simulink model "simu_py"  (R2025b)
settings: Solver=ode8  StartTime=0.0  StopTime=5  FixedStep=0.001  RelTol=1e-3
libraries: autolibshared x1
(part 2 of 2)

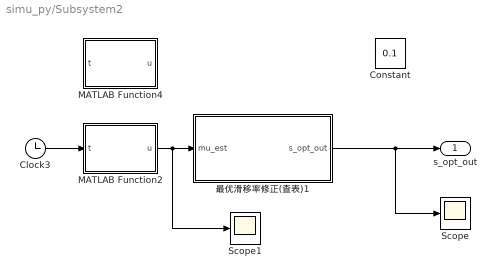
== system simu_py/Subsystem2 ==
  Clock3 : Clock
  Constant : Constant  Value=0.1
  MATLAB Function2 : MATLAB Function  TreatAsAtomicUnit=on
  MATLAB Function4 : MATLAB Function  TreatAsAtomicUnit=on
  Scope : Scope
      settings: ActiveDisplayYMinimum=0.051875  ActiveDisplayYMaximum=0.183125  DataLoggingVariableName=lambda_ref  DataLoggingSaveFormat=Array
  Scope1 : Scope
      settings: DataLoggingVariableName=mu_rel  DataLoggingSaveFormat=Array
  最优滑移率修正(查表)1 : MATLAB Function  TreatAsAtomicUnit=on
  s_opt_out : Outport
  wires:
  最优滑移率修正(查表)1/1(s_opt_out) -> s_opt_out/1, Scope/1
  MATLAB Function2/1(u) -> Scope1/1, 最优滑移率修正(查表)1/1(mu_est)
  Clock3/1 -> MATLAB Function2/1(t)

== matlab function simu_py/MATLAB Function17 ==
  data: mu_init input; c1_out output; c2_out output; c3_out output
function [c1_out, c2_out, c3_out] = select_initial_c(mu_init)
% 输入：
%   mu_init - 初始路面峰值附着系数（标量）
% 输出：
%   c1_out, c2_out, c3_out - 表中差值最小行对应的 c1,c2,c3 （标量）
%
% 说明：表格格式为每行 [c1, c2, c3, s_opt, mu_max]

% 如果传入向量/数组，只取第一个元素（Simulink 通常给标量）
if isempty(mu_init)
    mu_init = 0;
end
mu_init = double(mu_init(1));

% ----- 参数表（硬编码） -----
% 每行： [c1, c2, c3, s_opt, mu_max]
tbl = [ ...
    0.05,  306.39, 0.001, 0.03, 0.05;
    0.195, 94.129, 0.065, 0.065,0.191;
    0.4,   33.712, 0.12,  0.13, 0.4;
    0.857, 33.822, 0.35,  0.14, 0.8;
    1.197, 25.166, 0.54,  0.16, 1.09;
    1.281, 23.992, 0.52,  0.17, 1.17];

% ----- 计算与返回 -----
mu_table = tbl(:,5);            % 表中 mu_max 列
[~, idx] = min(abs(mu_table - mu_init)); % 找到差值最小的行（首个最小）
c1_out = tbl(idx,1);
c2_out = tbl(idx,2);
c3_out = tbl(idx,3);
end

== matlab function simu_py/MATLAB Function3 ==
  data: t input; u output
function u = fcn(t)
if t<1.5
    u=1.09;
elseif t>=1.5&&t<2.8
    u = 0.15;
elseif t>=2.8&&t<3.3
    u = 0.9;
elseif t>=3.3&&t<4.1
    u = 0.45;
else
    u = 0.9;
end

== matlab function simu_py/MATLAB Function6 ==
  data: t input; u output
function u = fcn(t)
if t<1.5
    u=1.09;
elseif t>=1.5&&t<2.8
    u = 0.15;
elseif t>=2.8&&t<3.3
    u = 0.9;
elseif t>=3.3&&t<4.1
    u = 0.45;
else
    u = 0.9;
end

== matlab function simu_py/MATLAB Function7 ==
  settings: updateMethod=DISCRETE
  data: Fz input; Td_out output; mu input; omega input; lambda_k input; lambda_ref input
function Td_out = OnlineFmincon_block(Fz, mu, omega, lambda_k, lambda_ref)
% Called inside Simulink MATLAB Function block
coder.extrinsic('my_sqp_nmpc_fix_tyretran.m'); % wrapper is extrinsic (run in MATLAB workspace)

% persistent state for initial guess
persistent Td
if isempty(Td)
    Td = zeros(4,1)+1;
end

% Call the MATLAB wrapper (extrinsic) - all args numeric (no function handles)
Td_opt = my_sqp_nmpc_fix_tyretran(Td, Fz, mu, omega, lambda_k, lambda_ref);

% Td_opt will be returned as a MATLAB array (extrinsic) - may need conversion
% assign back, output
if ~isempty(Td_opt)
    Td = Td_opt;
end

Td_out = Td;
end

== matlab function simu_py/Subsystem2/MATLAB Function2 ==
  data: t input; u output
function u = fcn(t)
if t<1.5
    u=1.09;
elseif t>=1.5&&t<2.8
    u = 0.15;
elseif t>=2.8&&t<3.3
    u = 0.9;
elseif t>=3.3&&t<4.1
    u = 0.45;
else
    u = 0.9;
end

== matlab function simu_py/Subsystem2/MATLAB Function4 ==
  data: t input; u output
function u = fcn(t)
if t<5
 u=0.85;
elseif t>=5 && t <10
    u = 0.3;
else
    u=1.09;
end
% elseif t>=5&&t<5.4
%    u=1.09-(t-5)*(1.09-0.2)/0.4;
% elseif t >= 5 && t<10
% %elseif t>=5.4&&t<10
%     u=0.2;
% %elseif t>=10&&t<11
% else
%     %u=0.2+(t-10)*(0.3-0.2)/1;
%     %u=0.2;
% % else 
%     u=0.2;
% end

== matlab function simu_py/Subsystem2/最优滑移率修正(查表)1 ==
  data: mu_est input; s_opt_out output
function s_opt_out = select_sopt_from_est(mu_est)
% 输入：
%   mu_est - 估计得到的路面峰值附着系数（标量）
% 输出：
%   s_opt_out - 从表中找到差值最小行对应的 s_opt（标量）
%
% 说明：表格格式为每行 [c1, c2, c3, s_opt, mu_max]

if isempty(mu_est)
    mu_est = 0;
end
mu_est = double(mu_est(1));

% ----- 参数表（硬编码，同上） -----
tbl = [ ...
    0.05,  306.39, 0.001, 0.03, 0.05;
    0.195, 94.129, 0.065, 0.065,0.191;
    0.4,   33.712, 0.12,  0.13, 0.4;
    0.857, 33.822, 0.35,  0.14, 0.8;
    1.197, 25.166, 0.54,  0.16, 1.09;
    1.281, 23.992, 0.52,  0.17, 1.17];

mu_table = tbl(:,5);
[~, idx] = min(abs(mu_table - mu_est));
s_opt_out = tbl(idx,4);
end

== matlab function simu_py/MATLAB Function8 ==
  settings: updateMethod=DISCRETE
  data: Td input; Fxf_hat output; dwm input; P_prev input; Pf_next output
function [Fxf_hat, Pf_next] = KF_TireForce(Td, dwm, P_prev)
% 一步卡尔曼滤波轮胎力估计
% 输入:
%   Td      -- 制动力矩输入 (Nm)
%   dwm     -- 观测到的角加速度 (rad/s^2)，含噪声
%   P_prev  -- 上一步的协方差
% 输出:
%   Fx_hat  -- 当前时刻估计的轮胎纵向力
%   P_next  -- 下一步更新后的协方差

% 固定参数 (可改为输入，或者用persistent存储)
J = 1.8;   % 转动惯量
r = 0.35;   % 车轮半径
H = -r/J;     % 观测矩阵
Q = 0.05;     % 过程噪声
R = 10;       % 测量噪声

% ---- 卡尔曼滤波步骤 ----
% 1. 先验估计 (状态转移 F=1, 无控制项)
Fx_prior = 0;  % 这里状态是“上一时刻Fx”，若要保持连续，可以persistent存储
persistent Fx_est
if isempty(Fx_est)
    Fx_est = 1200; % 初始估计
end
Fx_prior = Fx_est;

% 2. 协方差预测
P_prior = P_prev + Q;

% 3. 卡尔曼增益
Kk = P_prior*H / (H*P_prior*H + R);

% 4. 状态更新
% 观测方程: dwm ≈ (1/J)*(Td - r*Fx)
Fx_est = Fx_prior + Kk*(dwm - (1/J)*(Td - r*Fx_prior));

% 5. 协方差更新
Pf_next = (1 - Kk*H)*P_prior;

% 输出
Fxf_hat = Fx_est;
end

== matlab function simu_py/MATLAB Function9 ==
  settings: updateMethod=DISCRETE
  data: y input; s input; theta_out output; C1_0 input; C2_0 input; C3_0 input; P_out output; C1 output; C2 output; C3 output
function [theta_out, P_out, C1, C2,C3] = burckhardt_rnls(y, s,C1_0,C2_0,C3_0)
%y为轮胎力，s为滑移率
persistent theta P lambda eps_denom lb ub initialized
if isempty(initialized) 
    
    theta = [C1_0; C2_0; C3_0];

    % initial "covariance" P (large uncertainty)
    P = inv(1e-6*eye(3)); % tune per parameter scale

    % forgetting factor (0<lambda<=1). Closer to 1 -> slow forgetting.
    lambda = 0.995;

    % simple bounds for projection (prevent non-physical params)
    lb = [0.01; 10; 0.0];     % lower bounds for [C1; C2; C3]
    ub = [1.2; 350; 0.6];   % upper bounds

    initialized = true;
end


% --- compute model prediction at previous theta ---
C1 = theta(1);
C2 = theta(2);
C3 = theta(3);

% predicted mu at previous theta
yhat = C1*(1 - exp(-C2*s)) - C3*s;

% residual (current observation - prediction using previous theta)
r = y - yhat;

% --- compute Jacobian phi_k evaluated at previous theta ---
% phi = d(mu)/dtheta = [1 - exp(-C2*s); C1*s*exp(-C2*s); -s]
exp_term = exp(-C2*s);
phi = [1 - exp_term;
       C1 * s * exp_term;
       -s];

% --- RLS gain and update (Gauss-Newton style) ---
den = lambda + (phi' * (P * phi));

K = (P * phi) / den;   % 3x1 gain

% parameter update
theta = theta + K * r;

% projection (clip parameters to bounds)
%theta = max(lb, min(ub, theta));

% covariance update (RLS form)
I3 = eye(3);
P = (I3 - K * phi') * P / lambda;

% optional: ensure P remains symmetric positive definite numerically
%P = (P + P')/2;
% small floor on diagonal
%min_diag = 1e-9;
%for ii = 1:3
 %   if P(ii,ii) < min_diag
  %      P(ii,ii) = min_diag;
   % end
%end

% --- compute peak mu (analytic if possible, else numeric search) ---
C1 = theta(1); C2 = theta(2); C3 = theta(3);



% --- outputs ---
theta_out = theta;
P_out = norm(P);

end

== matlab function simu_py/MATLAB Function10 ==
  data: C1 input; C2 input; C3 input; mu_max output; iter output
function [mu_max, iter] = golden_max_burckhardt(C1, C2, C3)
% golden_max_burckhardt  在 [0, s_ub] 上用黄金分割法寻找 Burckhardt 模型的峰值
% mu(s) = C1*(1 - exp(-C2*s)) - C3*s
%
% 输入:
%   C1, C2, C3 - Burckhardt 参数 (标量)
%   tol        - 终止容差（区间长度阈值），例如 1e-6 （可选，默认1e-6）
%
% 输出:
%   s_star - 近似的使 mu 最大的 slip 点
%   mu_max - mu(s_star)
%   iter   - 迭代次数（实际执行的黄金分割步数）
%
% 说明:
%   - 优先尝试解析解: 解 dmu/ds = 0 得 s* = -1/C2 * log(C3/(C1*C2))，仅当 0<q<=1 时有效 (q=C3/(C1*C2))
%   - 若解析解不可用或不在 [0,s_ub] 内，则用黄金分割法在 [0,s_ub] 做数值搜索
%   - 代码包含数值保护，返回值受限为合理范围

% 默认参数
tol = 1e-6;

% 若未返回，则使用黄金分割法在 [0, s_ub] 搜索数值峰值
a = 0;
%搜索上界
b = 0.2;

% 黄金分割常数
gr = (sqrt(5) - 1) / 2;

% 初始化内点
c = b - gr * (b - a);
d = a + gr * (b - a);

fc = burckhardt_mu(c, C1, C2, C3);
fd = burckhardt_mu(d, C1, C2, C3);

maxit = 200;
for k = 1:maxit
    iter = k;
    % 因为寻找极大值，比较大小选择区间
    if fc > fd
        % 极大在左区间 [a, d]
        b = d;
        d = c;
        fd = fc;
        c = b - gr * (b - a);
        fc = burckhardt_mu(c, C1, C2, C3);
    else
        % 极大在右区间 [c, b]
        a = c;
        c = d;
        fc = fd;
        d = a + gr * (b - a);
        fd = burckhardt_mu(d, C1, C2, C3);
    end

    % 终止条件
    if (b - a) < tol
        break;
    end
end

% 结果取区间内 f 最大点 (c 或 d)
if fc > fd
    mu_max = fc;
else
    mu_max = fd;
end

if mu_max>1.13
    mu_max=1.13;
elseif mu_max<0.05
    mu_max=0.05;
end
end

% ---------- 辅助函数 ----------
function mu = burckhardt_mu(s, C1, C2, C3)
    % 计算 Burckhardt 模型的 mu(s)
    % 保护数值：确保 s 非负，避免 NaN
    s = double(max(0, s));
    % 直接计算
    mu = C1 * (1 - exp(-C2 * s)) - C3 * s;
end

== matlab function simu_py/最优滑移率修正(查表)2 ==
  data: mu_est input; s_opt_out output
function s_opt_out = select_sopt_from_est(mu_est)
% 输入：
%   mu_est - 估计得到的路面峰值附着系数（标量）
% 输出：
%   s_opt_out - 从表中找到差值最小行对应的 s_opt（标量）
%
% 说明：表格格式为每行 [c1, c2, c3, s_opt, mu_max]

if isempty(mu_est)
    mu_est = 0;
end
mu_est = double(mu_est(1));

% ----- 参数表（硬编码，同上） -----
tbl = [ ...
    0.05,  306.39, 0.001, 0.03, 0.05;
    0.195, 94.129, 0.065, 0.065,0.191;
    0.4,   33.712, 0.12,  0.13, 0.4;
    0.857, 33.822, 0.35,  0.14, 0.8;
    1.197, 25.166, 0.54,  0.16, 1.09;
    1.281, 23.992, 0.52,  0.17, 1.17];

mu_table = tbl(:,5);
[~, idx] = min(abs(mu_table - mu_est));
s_opt_out = tbl(idx,4);
end
